simulink model "flags_exec"  (Simulink 3.00)
libraries: execlib x5

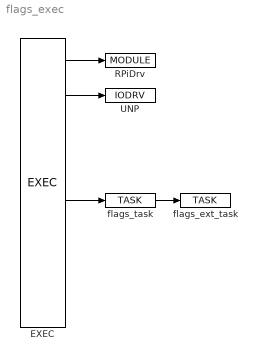
== system flags_exec ==
  EXEC : execlib/EXEC  target=Generic target device  tick=0.05  ntick0=10  ntick1=50  ntick2=100  ntick3=1200  pri0=5  pri1=9  pri2=13  pri3=18
  RPiDrv : execlib/MODULE
  UNP : execlib/IODRV  module=RPiDrv  classname=UnpDrv  factor=1  stack=10240  pri=3  timer=off
  flags_ext_task : execlib/TASK  factor=1  start=1  stop=2  stack=10240  MDLOPEN=on
  flags_task : execlib/TASK  factor=1  start=0  stop=1  stack=10240  MDLOPEN=on
  wires:
  EXEC/1 -> RPiDrv/1
  EXEC/2 -> UNP/1
  EXEC/5 -> flags_task/1
  flags_task/1 -> flags_ext_task/1
